simulink model "blance_leg"  (R2024a)
settings: Solver=VariableStepAuto  StartTime=0.0  StopTime=14  MaxStep=0.24  RelTol=1e-3
undefined symbols (not defined in the file): a11, a12, a13, a14, a15, a16, a21, a22, a23, a24, a25, a26, X, Y, Z
libraries: sm_lib x90, nesl_utility x22, matrix_library x4, slpidlib x2
(part 3 of 3)

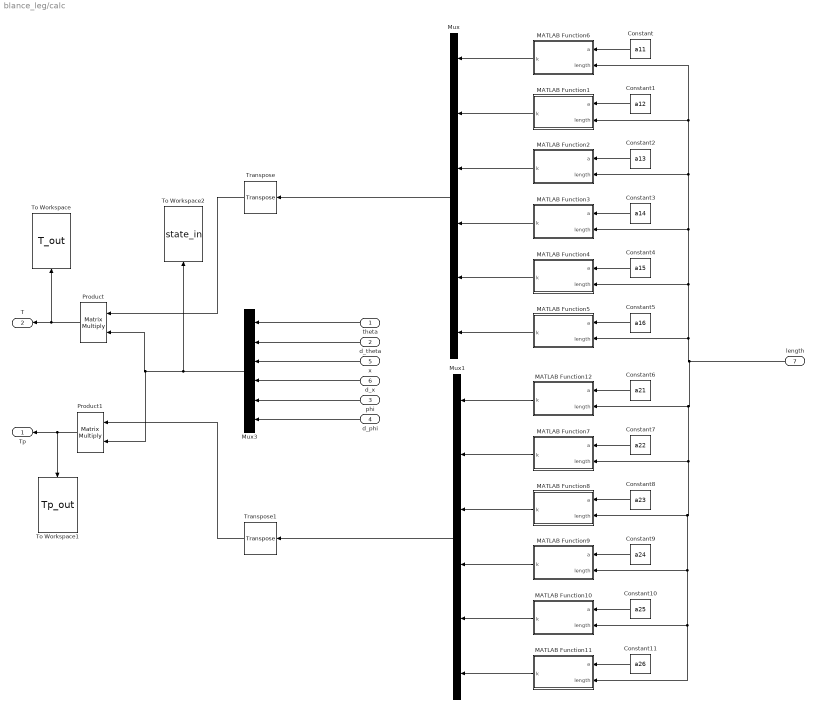
== system blance_leg/calc ==
  theta : Inport
  d_theta : Inport  Port=2
  phi : Inport  Port=3
  d_phi : Inport  Port=4
  x : Inport  Port=5
  d_x : Inport  Port=6
  length : Inport  Port=7
  Constant : Constant  Value=a11
  Constant1 : Constant  Value=a12
  Constant10 : Constant  Value=a25
  Constant11 : Constant  Value=a26
  Constant2 : Constant  Value=a13
  Constant3 : Constant  Value=a14
  Constant4 : Constant  Value=a15
  Constant5 : Constant  Value=a16
  Constant6 : Constant  Value=a21
  Constant7 : Constant  Value=a22
  Constant8 : Constant  Value=a23
  Constant9 : Constant  Value=a24
  MATLAB Function1 : MATLAB Function  TreatAsAtomicUnit=on
  MATLAB Function10 : MATLAB Function  TreatAsAtomicUnit=on
  MATLAB Function11 : MATLAB Function  TreatAsAtomicUnit=on
  MATLAB Function12 : MATLAB Function  TreatAsAtomicUnit=on
  MATLAB Function2 : MATLAB Function  TreatAsAtomicUnit=on
  MATLAB Function3 : MATLAB Function  TreatAsAtomicUnit=on
  MATLAB Function4 : MATLAB Function  TreatAsAtomicUnit=on
  MATLAB Function5 : MATLAB Function  TreatAsAtomicUnit=on
  MATLAB Function6 : MATLAB Function  TreatAsAtomicUnit=on
  MATLAB Function7 : MATLAB Function  TreatAsAtomicUnit=on
  MATLAB Function8 : MATLAB Function  TreatAsAtomicUnit=on
  MATLAB Function9 : MATLAB Function  TreatAsAtomicUnit=on
  Mux : Mux  Inputs=6
  Mux1 : Mux  Inputs=6
  Mux3 : Mux  Inputs=6
  Product : Product  Multiplication=Matrix(*)
  Product1 : Product  Multiplication=Matrix(*)
  To Workspace : ToWorkspace  VariableName=T_out  SampleTime=-1
      settings: Save2DSignal=2-D array (concatenate along first dimension)
  To Workspace1 : ToWorkspace  VariableName=Tp_out  SampleTime=-1
      settings: Save2DSignal=2-D array (concatenate along first dimension)
  To Workspace2 : ToWorkspace  VariableName=state_in  SampleTime=-1
      settings: Save2DSignal=2-D array (concatenate along first dimension)
  Transpose : matrix_library/Transpose
  Transpose1 : matrix_library/Transpose
  Tp : Outport
  T : Outport  Port=2
  wires:
  theta/1 -> Mux3/1
  d_theta/1 -> Mux3/2
  x/1 -> Mux3/3
  d_x/1 -> Mux3/4
  phi/1 -> Mux3/5
  d_phi/1 -> Mux3/6
  Constant/1 -> MATLAB Function6/1(a)
  Constant1/1 -> MATLAB Function1/1(a)
  Constant2/1 -> MATLAB Function2/1(a)
  Constant3/1 -> MATLAB Function3/1(a)
  Constant4/1 -> MATLAB Function4/1(a)
  Constant5/1 -> MATLAB Function5/1(a)
  Constant11/1 -> MATLAB Function11/1(a)
  Constant10/1 -> MATLAB Function10/1(a)
  Constant9/1 -> MATLAB Function9/1(a)
  Constant8/1 -> MATLAB Function8/1(a)
  Constant7/1 -> MATLAB Function7/1(a)
  Constant6/1 -> MATLAB Function12/1(a)
  MATLAB Function6/1(k) -> Mux/1
  MATLAB Function1/1(k) -> Mux/2
  MATLAB Function2/1(k) -> Mux/3
  MATLAB Function3/1(k) -> Mux/4
  MATLAB Function4/1(k) -> Mux/5
  MATLAB Function5/1(k) -> Mux/6
  MATLAB Function8/1(k) -> Mux1/3
  MATLAB Function11/1(k) -> Mux1/6
  MATLAB Function12/1(k) -> Mux1/1
  MATLAB Function7/1(k) -> Mux1/2
  MATLAB Function9/1(k) -> Mux1/4
  MATLAB Function10/1(k) -> Mux1/5
  length/1 -> MATLAB Function9/2(length), MATLAB Function10/2(length), MATLAB Function11/2(length), MATLAB Function8/2(length), MATLAB Function7/2(length), MATLAB Function12/2(length), MATLAB Function6/2(length), MATLAB Function1/2(length), MATLAB Function2/2(length), MATLAB Function3/2(length), MATLAB Function4/2(length), MATLAB Function5/2(length)
  Mux3/1 -> To Workspace2/1, Product1/2, Product/2
  Product1/1 -> Tp/1, To Workspace1/1
  Product/1 -> To Workspace/1, T/1
  Mux/1 -> Transpose/1
  Mux1/1 -> Transpose1/1
  Transpose/1 -> Product/1
  Transpose1/1 -> Product1/1

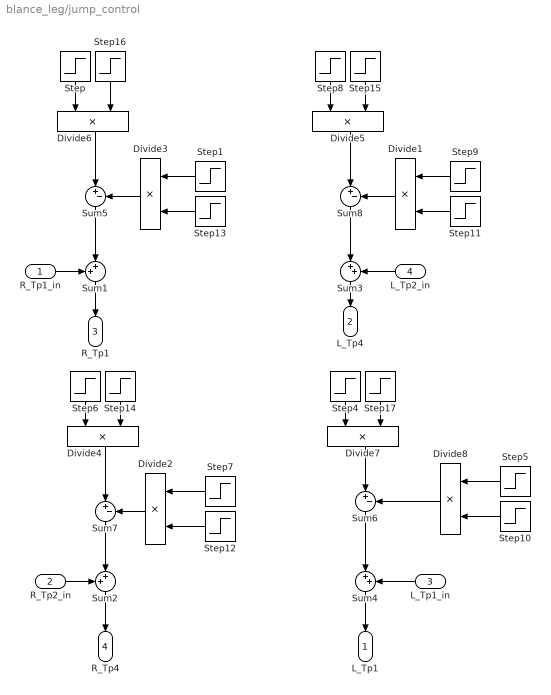
== system blance_leg/jump_control ==
  R_Tp1_in : Inport
  R_Tp2_in : Inport  Port=2
  L_Tp1_in : Inport  Port=3
  L_Tp2_in : Inport  Port=4
  Divide{1..8} (8 alike) : Product  Inputs=**
  Step : Step  Time=jump_time  After=-35  SampleTime=0
  Step1 : Step  Time=jump_time+0.15  After=-30  SampleTime=0
  Step{10..13} (4 alike) : Step  Time=jump_time+0.4  Before=1  After=0  SampleTime=0
  Step{14..17} (4 alike) : Step  Time=jump_time+0.2  Before=1  After=0  SampleTime=0
  Step4 : Step  Time=jump_time  After=-35  SampleTime=0
  Step5 : Step  Time=jump_time+0.15  After=-30  SampleTime=0
  Step6 : Step  Time=jump_time  After=35  SampleTime=0
  Step7 : Step  Time=jump_time+0.15  After=30  SampleTime=0
  Step8 : Step  Time=jump_time  After=35  SampleTime=0
  Step9 : Step  Time=jump_time+0.15  After=30  SampleTime=0
  Sum1 : Sum  Inputs=++|
  Sum2 : Sum  Inputs=++|
  Sum3 : Sum  Inputs=|++
  Sum4 : Sum  Inputs=|++
  Sum{5..8} (4 alike) : Sum  Inputs=|+-
  L_Tp1 : Outport
  L_Tp4 : Outport  Port=2
  R_Tp1 : Outport  Port=3
  R_Tp4 : Outport  Port=4
  wires:
  Divide4/1 -> Sum7/1
  Sum6/1 -> Sum4/1
  Step9/1 -> Divide1/1
  Step11/1 -> Divide1/2
  L_Tp1_in/1 -> Sum4/2
  Step1/1 -> Divide3/1
  Sum5/1 -> Sum1/2
  Step8/1 -> Divide5/1
  Step16/1 -> Divide6/2
  Divide3/1 -> Sum5/2
  Divide6/1 -> Sum5/1
  Step13/1 -> Divide3/2
  L_Tp2_in/1 -> Sum3/2
  Sum8/1 -> Sum3/1
  Step15/1 -> Divide5/2
  Step/1 -> Divide6/1
  Sum7/1 -> Sum2/2
  Divide5/1 -> Sum8/1
  Sum4/1 -> L_Tp1/1
  Sum2/1 -> R_Tp4/1
  Sum1/1 -> R_Tp1/1
  R_Tp2_in/1 -> Sum2/1
  R_Tp1_in/1 -> Sum1/1
  Sum3/1 -> L_Tp4/1
  Divide2/1 -> Sum7/2
  Step14/1 -> Divide4/2
  Step6/1 -> Divide4/1
  Step7/1 -> Divide2/1
  Step12/1 -> Divide2/2
  Divide1/1 -> Sum8/2
  Divide7/1 -> Sum6/1
  Step17/1 -> Divide7/2
  Step4/1 -> Divide7/1
  Divide8/1 -> Sum6/2
  Step10/1 -> Divide8/2
  Step5/1 -> Divide8/1

== matlab function blance_leg/calc/MATLAB Function12 ==
  data: k output; a input; length input
function k = get_K(a,length)
   k = polyval(a,length);  
end

== matlab function blance_leg/calc/MATLAB Function7 ==
  data: k output; a input; length input
function k = get_K(a,length)
   k = polyval(a,length);  
end

== matlab function blance_leg/calc/MATLAB Function8 ==
  data: k output; a input; length input
function k = get_K(a,length)
   k = polyval(a,length);  
end

== matlab function blance_leg/calc/MATLAB Function9 ==
  data: k output; a input; length input
function k = get_K(a,length)
   k = polyval(a,length);  
end

== matlab function blance_leg/calc/MATLAB Function6 ==
  data: k output; a input; length input
function k = get_K(a,length)
   k = polyval(a,length);  
end

== matlab function blance_leg/MATLAB Function7 ==
  data: L0 output; phi1 input; phi4 input
function L0  = L0(phi1,phi4)
   l5=0.108;
    l1=0.15;
    l2=0.25;
    l3=0.25;
    l4=0.15;
    YD = l4*sin(phi4);
    YB = l1*sin(phi1);
    XD = l5 + l4*cos(phi4);
    XB = l1*cos(phi1); 
    lBD = sqrt((XD - XB)*(XD - XB) + (YD - YB)*(YD - YB));
    A0 = 2*l2*(XD - XB);
    B0 = 2*l2*(YD - YB);
    C0 = l2*l2 + lBD*lBD - l3*l3;
    phi2 = 2*atan2((B0 + sqrt(A0*A0 + B0*B0 - C0*C0)),(A0 + C0));
    XC = l1*cos(phi1) + l2*cos(phi2);
    YC = l1*sin(phi1) + l2*sin(phi2);
    L0 = sqrt((XC - l5/2)*(XC - l5/2) + YC*YC);
   
end

== matlab function blance_leg/Subsystem1/MATLAB Function1 ==
  data: k output; a input; length input
function k = get_K(a,length)
   k = polyval(a,length);  
end

== matlab function blance_leg/Subsystem1/MATLAB Function10 ==
  data: k output; a input; length input
function k = get_K(a,length)
   k = polyval(a,length);  
end

== matlab function blance_leg/Subsystem1/MATLAB Function11 ==
  data: k output; a input; length input
function k = get_K(a,length)
   k = polyval(a,length);  
end

== matlab function blance_leg/Subsystem1/MATLAB Function12 ==
  data: k output; a input; length input
function k = get_K(a,length)
   k = polyval(a,length);  
end

== matlab function blance_leg/Subsystem1/MATLAB Function2 ==
  data: k output; a input; length input
function k = get_K(a,length)
   k = polyval(a,length);  
end

== matlab function blance_leg/Subsystem1/MATLAB Function3 ==
  data: k output; a input; length input
function k = get_K(a,length)
   k = polyval(a,length);  
end

== matlab function blance_leg/Subsystem1/MATLAB Function4 ==
  data: k output; a input; length input
function k = get_K(a,length)
   k = polyval(a,length);  
end

== matlab function blance_leg/Subsystem1/MATLAB Function5 ==
  data: k output; a input; length input
function k = get_K(a,length)
   k = polyval(a,length);  
end

== matlab function blance_leg/Subsystem1/MATLAB Function6 ==
  data: k output; a input; length input
function k = get_K(a,length)
   k = polyval(a,length);  
end

== matlab function blance_leg/calc/MATLAB Function1 ==
  data: k output; a input; length input
function k = get_K(a,length)
   k = polyval(a,length);  
end

== matlab function blance_leg/Subsystem1/MATLAB Function7 ==
  data: k output; a input; length input
function k = get_K(a,length)
   k = polyval(a,length);  
end

== matlab function blance_leg/Subsystem1/MATLAB Function8 ==
  data: k output; a input; length input
function k = get_K(a,length)
   k = polyval(a,length);  
end

== matlab function blance_leg/Subsystem1/MATLAB Function9 ==
  data: k output; a input; length input
function k = get_K(a,length)
   k = polyval(a,length);  
end

== matlab function blance_leg/MATLAB Function1 ==
  data: L0 output; phi1 input; phi4 input
function L0  = L0(phi1,phi4)
   l5=0.108;
    l1=0.15;
    l2=0.25;
    l3=0.25;
    l4=0.15;
    YD = l4*sin(phi4);
    YB = l1*sin(phi1);
    XD = l5 + l4*cos(phi4);
    XB = l1*cos(phi1); 
    lBD = sqrt((XD - XB)*(XD - XB) + (YD - YB)*(YD - YB));
    A0 = 2*l2*(XD - XB);
    B0 = 2*l2*(YD - YB);
    C0 = l2*l2 + lBD*lBD - l3*l3;
    phi2 = 2*atan2((B0 + sqrt(A0*A0 + B0*B0 - C0*C0)),(A0 + C0));
    XC = l1*cos(phi1) + l2*cos(phi2);
    YC = l1*sin(phi1) + l2*sin(phi2);
    L0 = sqrt((XC - l5/2)*(XC - l5/2) + YC*YC);
   
end

== matlab function blance_leg/Controller/MATLAB Function1 ==
  data: J output; phi1 input; phi4 input
function J  = Jacobian(phi1,phi4)
    l5=0.108;
    l1=0.15;
    l2=0.25;
    l3=0.25;
    l4=0.15;
    YD = l4*sin(phi4);
    YB = l1*sin(phi1);
    XD = l5 + l4*cos(phi4);
    XB = l1*cos(phi1); 
    lBD = sqrt((XD - XB)*(XD - XB) + (YD - YB)*(YD - YB));
    A0 = 2*l2*(XD - XB);
    B0 = 2*l2*(YD - YB);
    C0 = l2*l2 + lBD*lBD - l3*l3;
    phi2 = 2*atan2((B0 + sqrt(A0*A0 + B0*B0 - C0*C0)),(A0 + C0));
    phi3 = atan2(YB-YD+l2*sin(phi2),XB-XD+l2*cos(phi2));
    XC = l1*cos(phi1) + l2*cos(phi2);
    YC = l1*sin(phi1) + l2*sin(phi2);
    L0 = sqrt((XC - l5/2)*(XC - l5/2) + YC*YC);
    phi0 = atan2(YC,XC - l5/2);

    j11 = (l1*sin(phi0-phi3)*sin(phi1-phi2))/sin(phi3-phi2);
    j12 = (l4*sin(phi0-phi2)*sin(phi3-phi4))/sin(phi3-phi2);
    j21 = (l1*cos(phi0-phi3)*sin(phi1-phi2))/(L0*sin(phi3-phi2));
    j22 = (l4*cos(phi0-phi2)*sin(phi3-phi4))/(L0*sin(phi3-phi2));
    J = [j11 j12; j21 j22];
end

== matlab function blance_leg/Controller/MATLAB Function2 ==
  data: F0 input; T1 output; Tp input; J input; T2 output
function [T1,T2] = VMC_calc(F0,Tp,J)
F = [F0;Tp];
T = (J.') * F;
T1 = T(1,1);
T2 = T(2,1);
end

== matlab function blance_leg/Controller/MATLAB Function3 ==
  data: d_phi0 output; J input; d_phi1 input; d_phi4 input
function d_phi0 = D_PHI0(J,d_phi1,d_phi4)
    d_phi0 = J(2,1)*d_phi1 +J(2,2)*d_phi4;
end
    % syms phi_0 phi_1 phi_2 phi_4 l1 l2 l3 l4 l5 L0 d_phi1 d_phi4
    % 
    % XD=l5+l4*cos(phi_4);
    % YD=l4*sin(phi_4);
    % XB=l1*cos(phi_1);
    % YB=l1*sin(phi_1);
    % A0=2*l2*(XD-XB);
    % B0=2*l2*(YD-YB);
    % lBD=sqrt((XD-XB)^2+(YD-YB)^2);
    % C0=l2^2+lBD^2-l3^2;
    % phi_2=2*atan((B0+sqrt(A0^2+B0^2-C0^2))/(A0+C0));
    % XC=XB+l2*cos(phi_2);
    % YC=YB+l2*sin(phi_2);
    % L0=sqrt((XC-l5/2)^2+YC^2);
    % phi_0=atan(YC/(XC-l5/2));
    % 
    % J=jacobian([L0;phi_0],[phi_1;phi_4]);
    % phi0_dot = J(2,1)*d_phi1 +J(2,2)*d_phi4

    % jacobian函数无法在simulink中使用，故直接使用jacobian函数的最终结果

== matlab function blance_leg/Controller1/MATLAB Function2 ==
  data: F0 input; T1 output; Tp input; J input; T2 output
function [T1,T2] = VMC_calc(F0,Tp,J)
F = [F0;Tp];
T = (J.') * F;
T1 = T(1,1);
T2 = T(2,1);
end

== matlab function blance_leg/Controller1/MATLAB Function3 ==
  data: d_phi0 output; J input; d_phi1 input; d_phi4 input
function d_phi0 = D_PHI0(J,d_phi1,d_phi4)
    d_phi0 = J(2,1)*d_phi1 +J(2,2)*d_phi4;
end
    % syms phi_0 phi_1 phi_2 phi_4 l1 l2 l3 l4 l5 L0 d_phi1 d_phi4
    % 
    % XD=l5+l4*cos(phi_4);
    % YD=l4*sin(phi_4);
    % XB=l1*cos(phi_1);
    % YB=l1*sin(phi_1);
    % A0=2*l2*(XD-XB);
    % B0=2*l2*(YD-YB);
    % lBD=sqrt((XD-XB)^2+(YD-YB)^2);
    % C0=l2^2+lBD^2-l3^2;
    % phi_2=2*atan((B0+sqrt(A0^2+B0^2-C0^2))/(A0+C0));
    % XC=XB+l2*cos(phi_2);
    % YC=YB+l2*sin(phi_2);
    % L0=sqrt((XC-l5/2)^2+YC^2);
    % phi_0=atan(YC/(XC-l5/2));
    % 
    % J=jacobian([L0;phi_0],[phi_1;phi_4]);
    % phi0_dot = J(2,1)*d_phi1 +J(2,2)*d_phi4

    % jacobian函数无法在simulink中使用，故直接使用jacobian函数的最终结果

== matlab function blance_leg/calc/MATLAB Function2 ==
  data: k output; a input; length input
function k = get_K(a,length)
   k = polyval(a,length);  
end

== matlab function blance_leg/calc/MATLAB Function3 ==
  data: k output; a input; length input
function k = get_K(a,length)
   k = polyval(a,length);  
end

== matlab function blance_leg/calc/MATLAB Function4 ==
  data: k output; a input; length input
function k = get_K(a,length)
   k = polyval(a,length);  
end

== matlab function blance_leg/calc/MATLAB Function5 ==
  data: k output; a input; length input
function k = get_K(a,length)
   k = polyval(a,length);  
end

== matlab function blance_leg/Controller/MATLAB Function10 ==
  data: L0 output; phi1 input; phi4 input; phi0 output
function [L0,phi0] = L0_PHI0(phi1,phi4)
    l5=0.108;
    l1=0.15;
    l2=0.25;
    l3=0.25;
    l4=0.15;
    YD = l4*sin(phi4);
    YB = l1*sin(phi1);
    XD = l5 + l4*cos(phi4);
    XB = l1*cos(phi1); 
    lBD = sqrt((XD - XB)*(XD - XB) + (YD - YB)*(YD - YB));
    A0 = 2*l2*(XD - XB);
    B0 = 2*l2*(YD - YB);
    C0 = l2*l2 + lBD*lBD - l3*l3;
    phi2 = 2*atan2((B0 + sqrt(A0*A0 + B0*B0 - C0*C0)),(A0 + C0));
    XC = l1*cos(phi1) + l2*cos(phi2);
    YC = l1*sin(phi1) + l2*sin(phi2);
    L0 = sqrt((XC - l5/2)*(XC - l5/2) + YC*YC);
    phi0=atan2(YC,(XC-l5/2));
    
end

== matlab function blance_leg/Controller1/MATLAB Function1 ==
  data: J output; phi1 input; phi4 input
function J  = Jacobian(phi1,phi4)
    l5=0.108;
    l1=0.15;
    l2=0.25;
    l3=0.25;
    l4=0.15;
    YD = l4*sin(phi4);
    YB = l1*sin(phi1);
    XD = l5 + l4*cos(phi4);
    XB = l1*cos(phi1); 
    lBD = sqrt((XD - XB)*(XD - XB) + (YD - YB)*(YD - YB));
    A0 = 2*l2*(XD - XB);
    B0 = 2*l2*(YD - YB);
    C0 = l2*l2 + lBD*lBD - l3*l3;
    phi2 = 2*atan2((B0 + sqrt(A0*A0 + B0*B0 - C0*C0)),(A0 + C0));
    phi3 = atan2(YB-YD+l2*sin(phi2),XB-XD+l2*cos(phi2));
    XC = l1*cos(phi1) + l2*cos(phi2);
    YC = l1*sin(phi1) + l2*sin(phi2);
    L0 = sqrt((XC - l5/2)*(XC - l5/2) + YC*YC);
    phi0 = atan2(YC,XC - l5/2);

    j11 = (l1*sin(phi0-phi3)*sin(phi1-phi2))/sin(phi3-phi2);
    j12 = (l4*sin(phi0-phi2)*sin(phi3-phi4))/sin(phi3-phi2);
    j21 = (l1*cos(phi0-phi3)*sin(phi1-phi2))/(L0*sin(phi3-phi2));
    j22 = (l4*cos(phi0-phi2)*sin(phi3-phi4))/(L0*sin(phi3-phi2));
    J = [j11 j12; j21 j22];
end

== matlab function blance_leg/Controller1/MATLAB Function10 ==
  data: L0 output; phi1 input; phi4 input; phi0 output
function [L0,phi0] = L0_PHI0(phi1,phi4)
    l5=0.108;
    l1=0.15;
    l2=0.25;
    l3=0.25;
    l4=0.15;
    YD = l4*sin(phi4);
    YB = l1*sin(phi1);
    XD = l5 + l4*cos(phi4);
    XB = l1*cos(phi1); 
    lBD = sqrt((XD - XB)*(XD - XB) + (YD - YB)*(YD - YB));
    A0 = 2*l2*(XD - XB);
    B0 = 2*l2*(YD - YB);
    C0 = l2*l2 + lBD*lBD - l3*l3;
    phi2 = 2*atan2((B0 + sqrt(A0*A0 + B0*B0 - C0*C0)),(A0 + C0));
    XC = l1*cos(phi1) + l2*cos(phi2);
    YC = l1*sin(phi1) + l2*sin(phi2);
    L0 = sqrt((XC - l5/2)*(XC - l5/2) + YC*YC);
    phi0=atan2(YC,(XC-l5/2));
    
end

== matlab function blance_leg/calc/MATLAB Function10 ==
  data: k output; a input; length input
function k = get_K(a,length)
   k = polyval(a,length);  
end

== matlab function blance_leg/calc/MATLAB Function11 ==
  data: k output; a input; length input
function k = get_K(a,length)
   k = polyval(a,length);  
end
